simulink model "Neigungswinkel"  (R2019a)
settings: Solver=FixedStepAuto  StartTime=0.0  StopTime=inf  FixedStep=Ts  RelTol=1e-3  EnableMultiTasking=on
undefined symbols (not defined in the file): DiscIntNeverNeededParam, Ts
settings Model: SimulationMode=external  Creator=christinefux  LastModifiedBy=florian
settings SolverCC: PositivePriorityOrder=on
settings OptimizationCC: EnhancedBackFolding=on  PassReuseOutputArgsAs=Individual arguments  MaxStackSize=64  OptimizeBlockOrder=speed  DifferentSizesBufferReuse=on  OptimizationCustomize=off
settings DebuggingCC: ParameterTunabilityLossMsg=error
settings HardwareCC: ProdBitPerPointer=32  ProdBitPerSizeT=32  ProdBitPerPtrDiffT=32  ProdLargestAtomicInteger=Long  ProdLargestAtomicFloat=Double  ProdWordSize=32  ProdLongLongMode=on  ProdHWDeviceType=ARM Compatible->ARM Cortex
settings SFSimCC: MATLABDynamicMemAlloc=off
settings RTWCC: SystemTargetFile=ert.tlc  HardwareBoard=Raspberry Pi  TLCOptions="-aInlineSetEventsForThisBaseRateFcn=TLC_FALSE -aSuppressMultiTaskScheduler=TLC_FALSE  -aRateBasedStepFcn=0"  TemplateMakefile=ert_default_tmf  GenerateReport=on  Toolchain=GNU GCC Raspberry Pi  IncludeHyperlinkInReport=on  LaunchReport=on  GenerateTraceInfo=on  GenerateTraceReport=on  GenerateTraceReportSl=on  GenerateTraceReportSf=on  GenerateTraceReportEml=on
settings CodeAppCC: ForceParamTrailComments=on  IgnoreCustomStorageClasses=off  OperatorAnnotations=on  SimulinkDataObjDesc=on  SFDataObjDesc=on  InsertBlockDesc=on
settings ERTTargetCC: SupportContinuousTime=on  SupportVariableSizeSignals=on

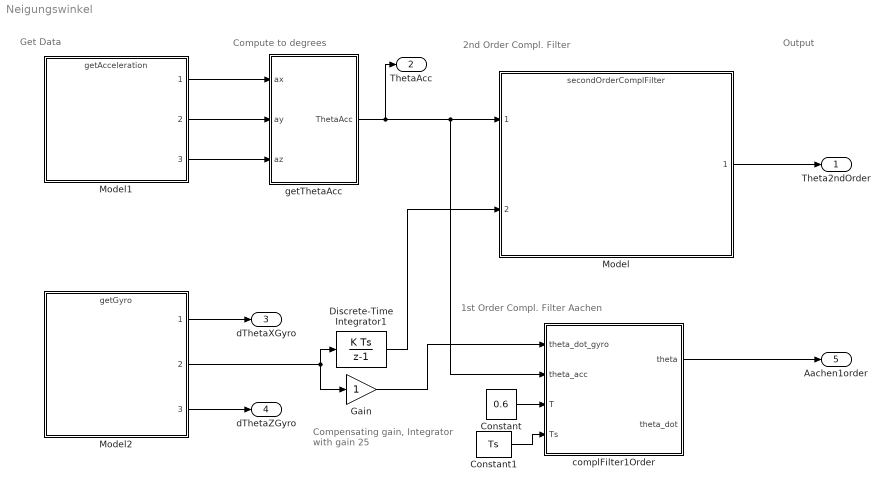
== system Neigungswinkel ==
  note: Output
  note: Compute to degrees
  note: Get Data
  note: 1st Order Compl. Filter Aachen
  note: 2nd Order Compl. Filter
  note: Compensating gain,
      | Integrator with gain 25
  Constant : Constant  Value=0.6
  Constant1 : Constant  Value=Ts
  Discrete-Time Integrator1 : DiscreteIntegrator  gainval=1  SampleTime=-1  ICPrevOutput=DiscIntNeverNeededParam  ICPrevScaledInput=DiscIntNeverNeededParam
  Gain : Gain
  Model : ModelReference  ModelNameDialog=secondOrderComplFilter.slx  SimulationMode=Normal  ModelReferenceVersion=1.18
  Model1 : ModelReference  ModelNameDialog=getAcceleration.slx  SimulationMode=Normal  ModelReferenceVersion=1.18
  Model2 : ModelReference  ModelNameDialog=getGyro.slx  SimulationMode=Normal  ModelReferenceVersion=1.25
  complFilter1Order : MATLAB Function  TreatAsAtomicUnit=on
  getThetaAcc : MATLAB Function  TreatAsAtomicUnit=on
  Theta2ndOrder : Outport
  ThetaAcc : Outport  Port=2
  dThetaXGyro : Outport  Port=3
  dThetaZGyro : Outport  Port=4
  Aachen1order : Outport  Port=5
  wires:
  getThetaAcc/1(ThetaAcc) -> ThetaAcc/1, Model/1, complFilter1Order/2(theta_acc)
  Model/1 -> Theta2ndOrder/1
  Model1/3 -> getThetaAcc/3(az)
  Model1/2 -> getThetaAcc/2(ay)
  Model1/1 -> getThetaAcc/1(ax)
  Model2/1 -> dThetaXGyro/1
  Model2/3 -> dThetaZGyro/1
  Constant/1 -> complFilter1Order/3(T)
  Constant1/1 -> complFilter1Order/4(Ts)
  complFilter1Order/1(theta) -> Aachen1order/1
  Discrete-Time Integrator1/1 -> Model/2
  Model2/2 -> Gain/1, Discrete-Time Integrator1/1
  Gain/1 -> complFilter1Order/1(theta_dot_gyro)

== matlab function Neigungswinkel/getThetaAcc ==
  data: ax input; ThetaAcc output; ay input; az input
function ThetaAcc = fcn(ax, ay, az)

ThetaAccRad = -atan2(-az,sqrt(ay.^2+ax.^2));    %Winkel aus Beschleunigungen rechnen
ThetaAcc = ThetaAccRad * 180 / pi;              %Winkel in deg umrechnen

== matlab function Neigungswinkel/complFilter1Order ==
  data: theta_dot_gyro input; theta output; theta_acc input; T input; Ts input; theta_dot output
function [theta, theta_dot] = fcn(theta_dot_gyro, theta_acc, T, Ts)
persistent last_theta
if isempty(last_theta)
    last_theta = 0;
end
alpha = T/(Ts + T);

% Aktuellen Winkel schätzen (Komplementärfilter)
theta = alpha*(last_theta + theta_dot_gyro*Ts) + (1-alpha)*theta_acc;
theta_dot = (theta-last_theta)/Ts;

% Aktuelles theta in Speicher schreiben
last_theta = theta;
